simulink model "ES105A_StHlthSigNormn"  (R2013b)
settings: Solver=FixedStepDiscrete  SolverMode=SingleTasking  StartTime=0.0  StopTime=1  FixedStep=0.002  RelTol=1e-3
undefined symbols (not defined in the file): ARCHGLBPRM_FLOATZEROTHD_ULS_F32, CurrMeasCorrlnMaxErrCurr, CURRMOTSUMDIVBYZEROPROTNVAL_AMPR_F32, DIGTQDIVBYZEROPROTNVAL_HWNWTMTR_F32, DutyCycThermProtnDutyCycFildThd, EcuTMeasRngDiagcMax, EcuTMeasRngDiagcMin, EotLrngAuthyStrtLrn, FRICESTIMNDIVBYZEROPROTNVAL_HWNWTMTR_F32, HLTH0PERC_CNT_U08, HLTH100PERC_CNT_F32, HLTH100PERC_CNT_U08, HLTH50PERC_CNT_U08, HwTqCorrlnChATraSumSetFltThd, HwTqCorrlnChBTraSumSetFltThd, HWTQIDPTSIG_CNT_U08, MOTAG2MEAS_VALMAXERR_VOLTSQD_F32, MOTAG2MEAS_VALMINERR_VOLTSQD_F32, MOTAGCORRLN_MOTAGCORRLNERRTHD_MOTREVELEC_U0P16, MotDrvDiagcErrThd, MOTPOS2DIVBYZEROPROTNVAL2_VOLTSQD_F32, MOTPOS2DIVBYZEROPROTNVAL_VOLTSQD_F32, MOTPOSNERRDIVBYZEROPROTNVAL_MOTREV_U16, MOTPOSNERRZEROTHD_MOTREV_U0P16, NtcNr1, NtcSts1, PHAVLTGDIVBYZEROPROTNVAL_NANOSEC_F32, SigQlfr1, STHLTHSCAGFAC_CNT_F32, StHlthSigNormnAbsltMotPosDifStHlthDiagThd, StHlthSigNormnCurrMotSumStHlthDiagThd, StHlthSigNormnDigTqStHlthDiagThd, StHlthSigNormnDutyCycFltLimThd, StHlthSigNormnHiCtrlrT, StHlthSigNormnIdptSigStHlthSca, StHlthSigNormnLoCtrlrT, StHlthSigNormnMaxFricThd, StHlthSigNormnMinRackTrvlLim, StHlthSigNormnMotPosStHlthDiagThd, StHlthSigNormnMotVelCal, StHlthSigNormnPhaInfoStHlthDiagThd, StHlthSigNormnStHlthCorrlnErr, StHlthSigNormnStHlthCurrMotSum, StHlthSigNormnStHlthPhaInfo, StHlthSigNormnValMaxStHlthErr, StHlthSigNormnValMinStHlthErr, StHlthSigNormnWhlImbRejctnThd, SysGlbPrmMotPoleCnt, TSTHLTH0PERC_CNT_U08, u2, u3, u4, VLTGSTHLTH0PERC_CNT_U08
libraries: NxtrLim x39, simulink x33, NxtrAbslt x4
(part 8 of 10)

== system ES105A_StHlthSigNormn/StHlthSigNormn/UpdRawSig/Motor Position Error /AbsltMotPosABDifStHlth Calc/If Action Subsystem/If Action Subsystem1 ==
  MotAgABErrTerm : Inport
  Action Port : ActionPort  ActionType=else
  Constant3 : Constant  Value=STHLTHSCAGFAC_CNT_F32
  CopyRight2 : Subsystem  Description=|  mask(Copyright Information){none=on}
      | Copyright info block.                                               
      |                                                                     
      | Place copyright information at the top of every subsystem in design.
      mask prompts: none "No parameters"
      mask help: Place copyright information at the top of every subsystem in design.
      mask Display:
      | NxtrConf = 'Nexteer Confidential';
      | 
      | sys = bdroot; %handle for the current model ("system")
      | first = get_param(sys,'Created');
      | first = first(end-3:end);  %year is last four digits
      | 
      | last = get_param(sys,'LastModifiedDate');
      | if isempty(last)
      |     last = datestr(now,'yyyy');
      | else
      |     last = last(end-3:end);
      | end
      | 
      | if strcmp(first,last)
      |     fprintf('%s -- Copyright %s Nexteer',NxtrConf,first)
      | else
      |     fprintf('%s -- %s%s- %s Nexteer',NxtrConf,char(169),first,last)
      | end
  Data Store Read : DataStoreRead  DataStoreName=MotAgCorrlnErrThd
  Data Type Conversion : DataTypeConversion  OutDataTypeStr=uint8
  Divide : Product  Inputs=*/
  Divide by Zero Protection for Cal : Subsystem
  LimStat_f32 : NxtrLim/LimStat_f32  LoLim=STHLTHFLOATZEROVAL_ULS_F32  HiLim=STHLTHFLOATTWOFIFTYFIVEVAL_ULS_F32
      settings: AttributesFormatString=|
      | Low Limit: %<LoLim>
      | High Limit:%<HiLim>
  Product : Product
  Subtract : Sum  Inputs=+-
  AbsltMotPosABDiffStHlth : Outport
  wires:
  Data Store Read/1 -> Subtract/1
  Subtract/1 -> Divide/1
  Constant3/1 -> Product/2
  MotAgABErrTerm/1 -> Subtract/2
  Divide/1 -> Product/1
  Divide by Zero Protection for Cal/1(CorrlnDelta) -> Divide/2
  LimStat_f32/1 -> Data Type Conversion/1
  Data Type Conversion/1 -> AbsltMotPosABDiffStHlth/1
  Product/1 -> LimStat_f32/1

== system ES105A_StHlthSigNormn/StHlthSigNormn/UpdRawSig/Motor Position Error /AbsltMotPosABDifStHlth Calc/If Action Subsystem1/CopyRight2 ==

== system ES105A_StHlthSigNormn/StHlthSigNormn/UpdRawSig/Motor Position Error /AbsltMotPosACDifStHlth Calc/If Action Subsystem4/CopyRight2 ==

== system ES105A_StHlthSigNormn/StHlthSigNormn/UpdRawSig/Motor Position Error /AbsltMotPosACDifStHlth Calc/If Action Subsystem4/If Action Subsystem ==
  Action Port : ActionPort  ActionType=then
  Constant : Constant  Value=HLTH0PERC_CNT_U08  OutDataTypeStr=uint8
  CopyRight2 : Subsystem  Description=|  mask(Copyright Information){none=on}
      | Copyright info block.                                               
      |                                                                     
      | Place copyright information at the top of every subsystem in design.
      mask prompts: none "No parameters"
      mask help: Place copyright information at the top of every subsystem in design.
      mask Display:
      | NxtrConf = 'Nexteer Confidential';
      | 
      | sys = bdroot; %handle for the current model ("system")
      | first = get_param(sys,'Created');
      | first = first(end-3:end);  %year is last four digits
      | 
      | last = get_param(sys,'LastModifiedDate');
      | if isempty(last)
      |     last = datestr(now,'yyyy');
      | else
      |     last = last(end-3:end);
      | end
      | 
      | if strcmp(first,last)
      |     fprintf('%s -- Copyright %s Nexteer',NxtrConf,first)
      | else
      |     fprintf('%s -- %s%s- %s Nexteer',NxtrConf,char(169),first,last)
      | end
  AbsltMotPosACDiffStHlth : Outport
  wires:
  Constant/1 -> AbsltMotPosACDiffStHlth/1

== system ES105A_StHlthSigNormn/StHlthSigNormn/UpdRawSig/Motor Position Error /AbsltMotPosACDifStHlth Calc/If Action Subsystem4/If Action Subsystem1 ==
  MotAgACErrTerm : Inport
  Action Port : ActionPort  ActionType=else
  Constant3 : Constant  Value=STHLTHSCAGFAC_CNT_F32
  CopyRight2 : Subsystem  Description=|  mask(Copyright Information){none=on}
      | Copyright info block.                                               
      |                                                                     
      | Place copyright information at the top of every subsystem in design.
      mask prompts: none "No parameters"
      mask help: Place copyright information at the top of every subsystem in design.
      mask Display:
      | NxtrConf = 'Nexteer Confidential';
      | 
      | sys = bdroot; %handle for the current model ("system")
      | first = get_param(sys,'Created');
      | first = first(end-3:end);  %year is last four digits
      | 
      | last = get_param(sys,'LastModifiedDate');
      | if isempty(last)
      |     last = datestr(now,'yyyy');
      | else
      |     last = last(end-3:end);
      | end
      | 
      | if strcmp(first,last)
      |     fprintf('%s -- Copyright %s Nexteer',NxtrConf,first)
      | else
      |     fprintf('%s -- %s%s- %s Nexteer',NxtrConf,char(169),first,last)
      | end
  Data Store Read : DataStoreRead  DataStoreName=MotAgCorrlnErrThd
  Data Type Conversion : DataTypeConversion  OutDataTypeStr=uint8
  Divide : Product  Inputs=*/
  Divide by Zero Protection for Cal : Subsystem
  LimStat_f32 : NxtrLim/LimStat_f32  LoLim=STHLTHFLOATZEROVAL_ULS_F32  HiLim=STHLTHFLOATTWOFIFTYFIVEVAL_ULS_F32
      settings: AttributesFormatString=|
      | Low Limit: %<LoLim>
      | High Limit:%<HiLim>
  Product : Product
  Subtract : Sum  Inputs=+-
  AbsltMotPosACDiffStHlth : Outport
  wires:
  Data Store Read/1 -> Subtract/1
  Subtract/1 -> Divide/1
  Constant3/1 -> Product/2
  MotAgACErrTerm/1 -> Subtract/2
  Divide/1 -> Product/1
  Divide by Zero Protection for Cal/1(CorrlnDelta) -> Divide/2
  LimStat_f32/1 -> Data Type Conversion/1
  Product/1 -> LimStat_f32/1
  Data Type Conversion/1 -> AbsltMotPosACDiffStHlth/1

== system ES105A_StHlthSigNormn/StHlthSigNormn/UpdRawSig/Motor Position Error /AbsltMotPosACDifStHlth Calc/If Action Subsystem5/CopyRight2 ==

== system ES105A_StHlthSigNormn/StHlthSigNormn/UpdRawSig/Motor Position Error /AbsltMotPosBCDifStHlth Calc/If Action Subsystem8/CopyRight2 ==

== system ES105A_StHlthSigNormn/StHlthSigNormn/UpdRawSig/Motor Position Error /AbsltMotPosBCDifStHlth Calc/If Action Subsystem8/If Action Subsystem ==
  Action Port : ActionPort  ActionType=then
  Constant : Constant  Value=HLTH0PERC_CNT_U08  OutDataTypeStr=uint8
  CopyRight2 : Subsystem  Description=|  mask(Copyright Information){none=on}
      | Copyright info block.                                               
      |                                                                     
      | Place copyright information at the top of every subsystem in design.
      mask prompts: none "No parameters"
      mask help: Place copyright information at the top of every subsystem in design.
      mask Display:
      | NxtrConf = 'Nexteer Confidential';
      | 
      | sys = bdroot; %handle for the current model ("system")
      | first = get_param(sys,'Created');
      | first = first(end-3:end);  %year is last four digits
      | 
      | last = get_param(sys,'LastModifiedDate');
      | if isempty(last)
      |     last = datestr(now,'yyyy');
      | else
      |     last = last(end-3:end);
      | end
      | 
      | if strcmp(first,last)
      |     fprintf('%s -- Copyright %s Nexteer',NxtrConf,first)
      | else
      |     fprintf('%s -- %s%s- %s Nexteer',NxtrConf,char(169),first,last)
      | end
  AbsltMotPosBCDiffStHlth : Outport
  wires:
  Constant/1 -> AbsltMotPosBCDiffStHlth/1

== system ES105A_StHlthSigNormn/StHlthSigNormn/UpdRawSig/Motor Position Error /AbsltMotPosBCDifStHlth Calc/If Action Subsystem8/If Action Subsystem1 ==
  MotAgBCErrTerm : Inport
  Action Port : ActionPort  ActionType=else
  Constant3 : Constant  Value=STHLTHSCAGFAC_CNT_F32
  CopyRight2 : Subsystem  Description=|  mask(Copyright Information){none=on}
      | Copyright info block.                                               
      |                                                                     
      | Place copyright information at the top of every subsystem in design.
      mask prompts: none "No parameters"
      mask help: Place copyright information at the top of every subsystem in design.
      mask Display:
      | NxtrConf = 'Nexteer Confidential';
      | 
      | sys = bdroot; %handle for the current model ("system")
      | first = get_param(sys,'Created');
      | first = first(end-3:end);  %year is last four digits
      | 
      | last = get_param(sys,'LastModifiedDate');
      | if isempty(last)
      |     last = datestr(now,'yyyy');
      | else
      |     last = last(end-3:end);
      | end
      | 
      | if strcmp(first,last)
      |     fprintf('%s -- Copyright %s Nexteer',NxtrConf,first)
      | else
      |     fprintf('%s -- %s%s- %s Nexteer',NxtrConf,char(169),first,last)
      | end
  Data Store Read : DataStoreRead  DataStoreName=MotAgCorrlnErrThd
  Data Type Conversion : DataTypeConversion  OutDataTypeStr=uint8
  Divide : Product  Inputs=*/
  Divide by Zero Protection for Cal : Subsystem
  LimStat_f32 : NxtrLim/LimStat_f32  LoLim=STHLTHFLOATZEROVAL_ULS_F32  HiLim=STHLTHFLOATTWOFIFTYFIVEVAL_ULS_F32
      settings: AttributesFormatString=|
      | Low Limit: %<LoLim>
      | High Limit:%<HiLim>
  Product : Product
  Subtract : Sum  Inputs=+-
  AbsltMotPosBCDiffStHlth : Outport
  wires:
  Data Store Read/1 -> Subtract/1
  Subtract/1 -> Divide/1
  Constant3/1 -> Product/2
  MotAgBCErrTerm/1 -> Subtract/2
  Divide/1 -> Product/1
  Divide by Zero Protection for Cal/1(CorrlnDelta) -> Divide/2
  LimStat_f32/1 -> Data Type Conversion/1
  Data Type Conversion/1 -> AbsltMotPosBCDiffStHlth/1
  Product/1 -> LimStat_f32/1

== system ES105A_StHlthSigNormn/StHlthSigNormn/UpdRawSig/Motor Position Error /AbsltMotPosBCDifStHlth Calc/If Action Subsystem9/CopyRight2 ==

== system ES105A_StHlthSigNormn/StHlthSigNormn/UpdRawSig/Motor Position Error /AbsltMotPosPhaDifStHlth/SetNtcSts/CopyRight2 ==

== system ES105A_StHlthSigNormn/StHlthSigNormn/UpdRawSig/Motor Position Error /NTC Sts Calculation/NtcFaild/CopyRight2 ==

== system ES105A_StHlthSigNormn/StHlthSigNormn/UpdRawSig/Motor Position Error /NTC Sts Calculation/NtcPassd/CopyRight2 ==

== system ES105A_StHlthSigNormn/StHlthSigNormn/UpdRawSig/Phase Voltage Verification/NTC Sts Calculation/NtcFaild/CopyRight2 ==

== system ES105A_StHlthSigNormn/StHlthSigNormn/UpdRawSig/Phase Voltage Verification/NTC Sts Calculation/NtcPassd/CopyRight2 ==

== system ES105A_StHlthSigNormn/StHlthSigNormn/UpdRawSig/Phase Voltage Verification/PhaAStHlth Calc/If Action Subsystem/CopyRight2 ==

== system ES105A_StHlthSigNormn/StHlthSigNormn/UpdRawSig/Phase Voltage Verification/PhaAStHlth Calc/If Action Subsystem/If Action Subsystem ==
  Action Port : ActionPort  ActionType=then
  Constant : Constant  Value=HLTH0PERC_CNT_U08  OutDataTypeStr=uint8
  CopyRight2 : Subsystem  Description=|  mask(Copyright Information){none=on}
      | Copyright info block.                                               
      |                                                                     
      | Place copyright information at the top of every subsystem in design.
      mask prompts: none "No parameters"
      mask help: Place copyright information at the top of every subsystem in design.
      mask Display:
      | NxtrConf = 'Nexteer Confidential';
      | 
      | sys = bdroot; %handle for the current model ("system")
      | first = get_param(sys,'Created');
      | first = first(end-3:end);  %year is last four digits
      | 
      | last = get_param(sys,'LastModifiedDate');
      | if isempty(last)
      |     last = datestr(now,'yyyy');
      | else
      |     last = last(end-3:end);
      | end
      | 
      | if strcmp(first,last)
      |     fprintf('%s -- Copyright %s Nexteer',NxtrConf,first)
      | else
      |     fprintf('%s -- %s%s- %s Nexteer',NxtrConf,char(169),first,last)
      | end
  PhaseAStHlth : Outport
  wires:
  Constant/1 -> PhaseAStHlth/1

== system ES105A_StHlthSigNormn/StHlthSigNormn/UpdRawSig/Phase Voltage Verification/PhaAStHlth Calc/If Action Subsystem/If Action Subsystem1 ==
  MotDrvErrA : Inport
  Action Port : ActionPort  ActionType=else
  Constant : Constant  Value=MotDrvDiagcErrThd
  Constant3 : Constant  Value=STHLTHSCAGFAC_CNT_F32
  CopyRight2 : Subsystem  Description=|  mask(Copyright Information){none=on}
      | Copyright info block.                                               
      |                                                                     
      | Place copyright information at the top of every subsystem in design.
      mask prompts: none "No parameters"
      mask help: Place copyright information at the top of every subsystem in design.
      mask Display:
      | NxtrConf = 'Nexteer Confidential';
      | 
      | sys = bdroot; %handle for the current model ("system")
      | first = get_param(sys,'Created');
      | first = first(end-3:end);  %year is last four digits
      | 
      | last = get_param(sys,'LastModifiedDate');
      | if isempty(last)
      |     last = datestr(now,'yyyy');
      | else
      |     last = last(end-3:end);
      | end
      | 
      | if strcmp(first,last)
      |     fprintf('%s -- Copyright %s Nexteer',NxtrConf,first)
      | else
      |     fprintf('%s -- %s%s- %s Nexteer',NxtrConf,char(169),first,last)
      | end
  Data Type Conversion : DataTypeConversion  OutDataTypeStr=uint8
  Divide : Product  Inputs=*/
  Divide by Zero Protection for Cal : Subsystem
  LimStat_f32 : NxtrLim/LimStat_f32  LoLim=STHLTHFLOATZEROVAL_ULS_F32  HiLim=STHLTHFLOATTWOFIFTYFIVEVAL_ULS_F32
      settings: AttributesFormatString=|
      | Low Limit: %<LoLim>
      | High Limit:%<HiLim>
  Product : Product
  Subtract : Sum  Inputs=+-
  PhaseAStHlth : Outport
  wires:
  Constant/1 -> Subtract/1
  MotDrvErrA/1 -> Subtract/2
  Subtract/1 -> Divide/1
  Constant3/1 -> Product/2
  Divide/1 -> Product/1
  Divide by Zero Protection for Cal/1(MotDrvDiagDelta) -> Divide/2
  LimStat_f32/1 -> Data Type Conversion/1
  Product/1 -> LimStat_f32/1
  Data Type Conversion/1 -> PhaseAStHlth/1

== system ES105A_StHlthSigNormn/StHlthSigNormn/UpdRawSig/Phase Voltage Verification/PhaAStHlth Calc/If Action Subsystem1/CopyRight2 ==

== system ES105A_StHlthSigNormn/StHlthSigNormn/UpdRawSig/Phase Voltage Verification/PhaBStHlth Calc/If Action Subsystem4/CopyRight2 ==

== system ES105A_StHlthSigNormn/StHlthSigNormn/UpdRawSig/Phase Voltage Verification/PhaBStHlth Calc/If Action Subsystem4/If Action Subsystem ==
  Action Port : ActionPort  ActionType=then
  Constant : Constant  Value=HLTH0PERC_CNT_U08  OutDataTypeStr=uint8
  CopyRight2 : Subsystem  Description=|  mask(Copyright Information){none=on}
      | Copyright info block.                                               
      |                                                                     
      | Place copyright information at the top of every subsystem in design.
      mask prompts: none "No parameters"
      mask help: Place copyright information at the top of every subsystem in design.
      mask Display:
      | NxtrConf = 'Nexteer Confidential';
      | 
      | sys = bdroot; %handle for the current model ("system")
      | first = get_param(sys,'Created');
      | first = first(end-3:end);  %year is last four digits
      | 
      | last = get_param(sys,'LastModifiedDate');
      | if isempty(last)
      |     last = datestr(now,'yyyy');
      | else
      |     last = last(end-3:end);
      | end
      | 
      | if strcmp(first,last)
      |     fprintf('%s -- Copyright %s Nexteer',NxtrConf,first)
      | else
      |     fprintf('%s -- %s%s- %s Nexteer',NxtrConf,char(169),first,last)
      | end
  PhaseBStHlth : Outport
  wires:
  Constant/1 -> PhaseBStHlth/1

== system ES105A_StHlthSigNormn/StHlthSigNormn/UpdRawSig/Phase Voltage Verification/PhaBStHlth Calc/If Action Subsystem4/If Action Subsystem1 ==
  MotDrvErrB : Inport
  Action Port : ActionPort  ActionType=else
  Constant : Constant  Value=MotDrvDiagcErrThd
  Constant3 : Constant  Value=STHLTHSCAGFAC_CNT_F32
  CopyRight2 : Subsystem  Description=|  mask(Copyright Information){none=on}
      | Copyright info block.                                               
      |                                                                     
      | Place copyright information at the top of every subsystem in design.
      mask prompts: none "No parameters"
      mask help: Place copyright information at the top of every subsystem in design.
      mask Display:
      | NxtrConf = 'Nexteer Confidential';
      | 
      | sys = bdroot; %handle for the current model ("system")
      | first = get_param(sys,'Created');
      | first = first(end-3:end);  %year is last four digits
      | 
      | last = get_param(sys,'LastModifiedDate');
      | if isempty(last)
      |     last = datestr(now,'yyyy');
      | else
      |     last = last(end-3:end);
      | end
      | 
      | if strcmp(first,last)
      |     fprintf('%s -- Copyright %s Nexteer',NxtrConf,first)
      | else
      |     fprintf('%s -- %s%s- %s Nexteer',NxtrConf,char(169),first,last)
      | end
  Data Type Conversion : DataTypeConversion  OutDataTypeStr=uint8
  Divide : Product  Inputs=*/
  Divide by Zero Protection for Cal : Subsystem
  LimStat_f32 : NxtrLim/LimStat_f32  LoLim=STHLTHFLOATZEROVAL_ULS_F32  HiLim=STHLTHFLOATTWOFIFTYFIVEVAL_ULS_F32
      settings: AttributesFormatString=|
      | Low Limit: %<LoLim>
      | High Limit:%<HiLim>
  Product : Product
  Subtract : Sum  Inputs=+-
  PhaseBStHlth : Outport
  wires:
  Constant/1 -> Subtract/1
  MotDrvErrB/1 -> Subtract/2
  Subtract/1 -> Divide/1
  Constant3/1 -> Product/2
  Divide/1 -> Product/1
  Divide by Zero Protection for Cal/1(MotDrvDiagDelta) -> Divide/2
  LimStat_f32/1 -> Data Type Conversion/1
  Product/1 -> LimStat_f32/1
  Data Type Conversion/1 -> PhaseBStHlth/1

== system ES105A_StHlthSigNormn/StHlthSigNormn/UpdRawSig/Phase Voltage Verification/PhaBStHlth Calc/If Action Subsystem5/CopyRight2 ==

== system ES105A_StHlthSigNormn/StHlthSigNormn/UpdRawSig/Phase Voltage Verification/PhaCStHlth Calc/If Action Subsystem8/CopyRight2 ==

== system ES105A_StHlthSigNormn/StHlthSigNormn/UpdRawSig/Phase Voltage Verification/PhaCStHlth Calc/If Action Subsystem8/If Action Subsystem ==
  Action Port : ActionPort  ActionType=then
  Constant : Constant  Value=HLTH0PERC_CNT_U08  OutDataTypeStr=uint8
  CopyRight2 : Subsystem  Description=|  mask(Copyright Information){none=on}
      | Copyright info block.                                               
      |                                                                     
      | Place copyright information at the top of every subsystem in design.
      mask prompts: none "No parameters"
      mask help: Place copyright information at the top of every subsystem in design.
      mask Display:
      | NxtrConf = 'Nexteer Confidential';
      | 
      | sys = bdroot; %handle for the current model ("system")
      | first = get_param(sys,'Created');
      | first = first(end-3:end);  %year is last four digits
      | 
      | last = get_param(sys,'LastModifiedDate');
      | if isempty(last)
      |     last = datestr(now,'yyyy');
      | else
      |     last = last(end-3:end);
      | end
      | 
      | if strcmp(first,last)
      |     fprintf('%s -- Copyright %s Nexteer',NxtrConf,first)
      | else
      |     fprintf('%s -- %s%s- %s Nexteer',NxtrConf,char(169),first,last)
      | end
  PhaseCStHlth : Outport
  wires:
  Constant/1 -> PhaseCStHlth/1

== system ES105A_StHlthSigNormn/StHlthSigNormn/UpdRawSig/Phase Voltage Verification/PhaCStHlth Calc/If Action Subsystem8/If Action Subsystem1 ==
  MotDrvErrC : Inport
  Action Port : ActionPort  ActionType=else
  Constant : Constant  Value=MotDrvDiagcErrThd
  Constant3 : Constant  Value=STHLTHSCAGFAC_CNT_F32
  CopyRight2 : Subsystem  Description=|  mask(Copyright Information){none=on}
      | Copyright info block.                                               
      |                                                                     
      | Place copyright information at the top of every subsystem in design.
      mask prompts: none "No parameters"
      mask help: Place copyright information at the top of every subsystem in design.
      mask Display:
      | NxtrConf = 'Nexteer Confidential';
      | 
      | sys = bdroot; %handle for the current model ("system")
      | first = get_param(sys,'Created');
      | first = first(end-3:end);  %year is last four digits
      | 
      | last = get_param(sys,'LastModifiedDate');
      | if isempty(last)
      |     last = datestr(now,'yyyy');
      | else
      |     last = last(end-3:end);
      | end
      | 
      | if strcmp(first,last)
      |     fprintf('%s -- Copyright %s Nexteer',NxtrConf,first)
      | else
      |     fprintf('%s -- %s%s- %s Nexteer',NxtrConf,char(169),first,last)
      | end
  Data Type Conversion : DataTypeConversion  OutDataTypeStr=uint8
  Divide : Product  Inputs=*/
  Divide by Zero Protection for Cal : Subsystem
  LimStat_f32 : NxtrLim/LimStat_f32  LoLim=STHLTHFLOATZEROVAL_ULS_F32  HiLim=STHLTHFLOATTWOFIFTYFIVEVAL_ULS_F32
      settings: AttributesFormatString=|
      | Low Limit: %<LoLim>
      | High Limit:%<HiLim>
  Product : Product
  Subtract : Sum  Inputs=+-
  PhaseCStHlth : Outport
  wires:
  Constant/1 -> Subtract/1
  MotDrvErrC/1 -> Subtract/2
  Subtract/1 -> Divide/1
  Constant3/1 -> Product/2
  Divide/1 -> Product/1
  Divide by Zero Protection for Cal/1(MotDrvDiagDelta) -> Divide/2
  LimStat_f32/1 -> Data Type Conversion/1
  Product/1 -> LimStat_f32/1
  Data Type Conversion/1 -> PhaseCStHlth/1

== system ES105A_StHlthSigNormn/StHlthSigNormn/UpdRawSig/Phase Voltage Verification/PhaCStHlth Calc/If Action Subsystem9/CopyRight2 ==

== system ES105A_StHlthSigNormn/StHlthSigNormn/UpdRawSig/Phase Voltage Verification/PhaDStHlth Calc/If Action Subsystem12/CopyRight2 ==

== system ES105A_StHlthSigNormn/StHlthSigNormn/UpdRawSig/Phase Voltage Verification/PhaDStHlth Calc/If Action Subsystem12/If Action Subsystem ==
  Action Port : ActionPort  ActionType=then
  Constant : Constant  Value=HLTH0PERC_CNT_U08  OutDataTypeStr=uint8
  CopyRight2 : Subsystem  Description=|  mask(Copyright Information){none=on}
      | Copyright info block.                                               
      |                                                                     
      | Place copyright information at the top of every subsystem in design.
      mask prompts: none "No parameters"
      mask help: Place copyright information at the top of every subsystem in design.
      mask Display:
      | NxtrConf = 'Nexteer Confidential';
      | 
      | sys = bdroot; %handle for the current model ("system")
      | first = get_param(sys,'Created');
      | first = first(end-3:end);  %year is last four digits
      | 
      | last = get_param(sys,'LastModifiedDate');
      | if isempty(last)
      |     last = datestr(now,'yyyy');
      | else
      |     last = last(end-3:end);
      | end
      | 
      | if strcmp(first,last)
      |     fprintf('%s -- Copyright %s Nexteer',NxtrConf,first)
      | else
      |     fprintf('%s -- %s%s- %s Nexteer',NxtrConf,char(169),first,last)
      | end
  PhaseDStHlth : Outport
  wires:
  Constant/1 -> PhaseDStHlth/1

== system ES105A_StHlthSigNormn/StHlthSigNormn/UpdRawSig/Phase Voltage Verification/PhaDStHlth Calc/If Action Subsystem12/If Action Subsystem1 ==
  MotDrvErrD : Inport
  Action Port : ActionPort  ActionType=else
  Constant : Constant  Value=MotDrvDiagcErrThd
  Constant3 : Constant  Value=STHLTHSCAGFAC_CNT_F32
  CopyRight2 : Subsystem  Description=|  mask(Copyright Information){none=on}
      | Copyright info block.                                               
      |                                                                     
      | Place copyright information at the top of every subsystem in design.
      mask prompts: none "No parameters"
      mask help: Place copyright information at the top of every subsystem in design.
      mask Display:
      | NxtrConf = 'Nexteer Confidential';
      | 
      | sys = bdroot; %handle for the current model ("system")
      | first = get_param(sys,'Created');
      | first = first(end-3:end);  %year is last four digits
      | 
      | last = get_param(sys,'LastModifiedDate');
      | if isempty(last)
      |     last = datestr(now,'yyyy');
      | else
      |     last = last(end-3:end);
      | end
      | 
      | if strcmp(first,last)
      |     fprintf('%s -- Copyright %s Nexteer',NxtrConf,first)
      | else
      |     fprintf('%s -- %s%s- %s Nexteer',NxtrConf,char(169),first,last)
      | end
  Data Type Conversion : DataTypeConversion  OutDataTypeStr=uint8
  Divide : Product  Inputs=*/
  Divide by Zero Protection for Cal : Subsystem
  LimStat_f32 : NxtrLim/LimStat_f32  LoLim=STHLTHFLOATZEROVAL_ULS_F32  HiLim=STHLTHFLOATTWOFIFTYFIVEVAL_ULS_F32
      settings: AttributesFormatString=|
      | Low Limit: %<LoLim>
      | High Limit:%<HiLim>
  Product : Product
  Subtract : Sum  Inputs=+-
  PhaseDStHlth : Outport
  wires:
  Constant/1 -> Subtract/1
  MotDrvErrD/1 -> Subtract/2
  Subtract/1 -> Divide/1
  Constant3/1 -> Product/2
  Divide/1 -> Product/1
  Divide by Zero Protection for Cal/1(MotDrvDiagDelta) -> Divide/2
  LimStat_f32/1 -> Data Type Conversion/1
  Product/1 -> LimStat_f32/1
  Data Type Conversion/1 -> PhaseDStHlth/1

== system ES105A_StHlthSigNormn/StHlthSigNormn/UpdRawSig/Phase Voltage Verification/PhaDStHlth Calc/If Action Subsystem13/CopyRight2 ==

== system ES105A_StHlthSigNormn/StHlthSigNormn/UpdRawSig/Phase Voltage Verification/PhaEStHlth Calc/If Action Subsystem16/CopyRight2 ==

== system ES105A_StHlthSigNormn/StHlthSigNormn/UpdRawSig/Phase Voltage Verification/PhaEStHlth Calc/If Action Subsystem16/If Action Subsystem ==
  Action Port : ActionPort  ActionType=then
  Constant : Constant  Value=HLTH0PERC_CNT_U08  OutDataTypeStr=uint8
  CopyRight2 : Subsystem  Description=|  mask(Copyright Information){none=on}
      | Copyright info block.                                               
      |                                                                     
      | Place copyright information at the top of every subsystem in design.
      mask prompts: none "No parameters"
      mask help: Place copyright information at the top of every subsystem in design.
      mask Display:
      | NxtrConf = 'Nexteer Confidential';
      | 
      | sys = bdroot; %handle for the current model ("system")
      | first = get_param(sys,'Created');
      | first = first(end-3:end);  %year is last four digits
      | 
      | last = get_param(sys,'LastModifiedDate');
      | if isempty(last)
      |     last = datestr(now,'yyyy');
      | else
      |     last = last(end-3:end);
      | end
      | 
      | if strcmp(first,last)
      |     fprintf('%s -- Copyright %s Nexteer',NxtrConf,first)
      | else
      |     fprintf('%s -- %s%s- %s Nexteer',NxtrConf,char(169),first,last)
      | end
  PhaseEStHlth : Outport
  wires:
  Constant/1 -> PhaseEStHlth/1

== system ES105A_StHlthSigNormn/StHlthSigNormn/UpdRawSig/Phase Voltage Verification/PhaEStHlth Calc/If Action Subsystem16/If Action Subsystem1 ==
  MotDrvErrE : Inport
  Action Port : ActionPort  ActionType=else
  Constant : Constant  Value=MotDrvDiagcErrThd
  Constant3 : Constant  Value=STHLTHSCAGFAC_CNT_F32
  CopyRight2 : Subsystem  Description=|  mask(Copyright Information){none=on}
      | Copyright info block.                                               
      |                                                                     
      | Place copyright information at the top of every subsystem in design.
      mask prompts: none "No parameters"
      mask help: Place copyright information at the top of every subsystem in design.
      mask Display:
      | NxtrConf = 'Nexteer Confidential';
      | 
      | sys = bdroot; %handle for the current model ("system")
      | first = get_param(sys,'Created');
      | first = first(end-3:end);  %year is last four digits
      | 
      | last = get_param(sys,'LastModifiedDate');
      | if isempty(last)
      |     last = datestr(now,'yyyy');
      | else
      |     last = last(end-3:end);
      | end
      | 
      | if strcmp(first,last)
      |     fprintf('%s -- Copyright %s Nexteer',NxtrConf,first)
      | else
      |     fprintf('%s -- %s%s- %s Nexteer',NxtrConf,char(169),first,last)
      | end
  Data Type Conversion : DataTypeConversion  OutDataTypeStr=uint8
  Divide : Product  Inputs=*/
  Divide by Zero Protection for Cal : Subsystem
  LimStat_f32 : NxtrLim/LimStat_f32  LoLim=STHLTHFLOATZEROVAL_ULS_F32  HiLim=STHLTHFLOATTWOFIFTYFIVEVAL_ULS_F32
      settings: AttributesFormatString=|
      | Low Limit: %<LoLim>
      | High Limit:%<HiLim>
  Product : Product
  Subtract : Sum  Inputs=+-
  PhaseEStHlth : Outport
  wires:
  Constant/1 -> Subtract/1
  MotDrvErrE/1 -> Subtract/2
  Subtract/1 -> Divide/1
  Constant3/1 -> Product/2
  Divide/1 -> Product/1
  Divide by Zero Protection for Cal/1(MotDrvDiagDelta) -> Divide/2
  LimStat_f32/1 -> Data Type Conversion/1
  Product/1 -> LimStat_f32/1
  Data Type Conversion/1 -> PhaseEStHlth/1

== system ES105A_StHlthSigNormn/StHlthSigNormn/UpdRawSig/Phase Voltage Verification/PhaEStHlth Calc/If Action Subsystem17/CopyRight2 ==

== system ES105A_StHlthSigNormn/StHlthSigNormn/UpdRawSig/Phase Voltage Verification/PhaFStHlth Calc/If Action Subsystem20/CopyRight2 ==

== system ES105A_StHlthSigNormn/StHlthSigNormn/UpdRawSig/Phase Voltage Verification/PhaFStHlth Calc/If Action Subsystem20/If Action Subsystem ==
  Action Port : ActionPort  ActionType=then
  Constant : Constant  Value=HLTH0PERC_CNT_U08  OutDataTypeStr=uint8
  CopyRight2 : Subsystem  Description=|  mask(Copyright Information){none=on}
      | Copyright info block.                                               
      |                                                                     
      | Place copyright information at the top of every subsystem in design.
      mask prompts: none "No parameters"
      mask help: Place copyright information at the top of every subsystem in design.
      mask Display:
      | NxtrConf = 'Nexteer Confidential';
      | 
      | sys = bdroot; %handle for the current model ("system")
      | first = get_param(sys,'Created');
      | first = first(end-3:end);  %year is last four digits
      | 
      | last = get_param(sys,'LastModifiedDate');
      | if isempty(last)
      |     last = datestr(now,'yyyy');
      | else
      |     last = last(end-3:end);
      | end
      | 
      | if strcmp(first,last)
      |     fprintf('%s -- Copyright %s Nexteer',NxtrConf,first)
      | else
      |     fprintf('%s -- %s%s- %s Nexteer',NxtrConf,char(169),first,last)
      | end
  PhaseFStHlth : Outport
  wires:
  Constant/1 -> PhaseFStHlth/1

== system ES105A_StHlthSigNormn/StHlthSigNormn/UpdRawSig/Phase Voltage Verification/PhaFStHlth Calc/If Action Subsystem20/If Action Subsystem1 ==
  MotDrvErrF : Inport
  Action Port : ActionPort  ActionType=else
  Constant : Constant  Value=MotDrvDiagcErrThd
  Constant3 : Constant  Value=STHLTHSCAGFAC_CNT_F32
  CopyRight2 : Subsystem  Description=|  mask(Copyright Information){none=on}
      | Copyright info block.                                               
      |                                                                     
      | Place copyright information at the top of every subsystem in design.
      mask prompts: none "No parameters"
      mask help: Place copyright information at the top of every subsystem in design.
      mask Display:
      | NxtrConf = 'Nexteer Confidential';
      | 
      | sys = bdroot; %handle for the current model ("system")
      | first = get_param(sys,'Created');
      | first = first(end-3:end);  %year is last four digits
      | 
      | last = get_param(sys,'LastModifiedDate');
      | if isempty(last)
      |     last = datestr(now,'yyyy');
      | else
      |     last = last(end-3:end);
      | end
      | 
      | if strcmp(first,last)
      |     fprintf('%s -- Copyright %s Nexteer',NxtrConf,first)
      | else
      |     fprintf('%s -- %s%s- %s Nexteer',NxtrConf,char(169),first,last)
      | end
  Data Type Conversion : DataTypeConversion  OutDataTypeStr=uint8
  Divide : Product  Inputs=*/
  Divide by Zero Protection for Cal : Subsystem
  LimStat_f32 : NxtrLim/LimStat_f32  LoLim=STHLTHFLOATZEROVAL_ULS_F32  HiLim=STHLTHFLOATTWOFIFTYFIVEVAL_ULS_F32
      settings: AttributesFormatString=|
      | Low Limit: %<LoLim>
      | High Limit:%<HiLim>
  Product : Product
  Subtract : Sum  Inputs=+-
  PhaseFStHlth : Outport
  wires:
  Constant/1 -> Subtract/1
  MotDrvErrF/1 -> Subtract/2
  Subtract/1 -> Divide/1
  Constant3/1 -> Product/2
  Divide/1 -> Product/1
  Divide by Zero Protection for Cal/1(MotDrvDiagDelta) -> Divide/2
  LimStat_f32/1 -> Data Type Conversion/1
  Product/1 -> LimStat_f32/1
  Data Type Conversion/1 -> PhaseFStHlth/1

== system ES105A_StHlthSigNormn/StHlthSigNormn/UpdRawSig/Phase Voltage Verification/PhaFStHlth Calc/If Action Subsystem21/CopyRight2 ==

== system ES105A_StHlthSigNormn/StHlthSigNormn/UpdRawSig/Phase Voltage Verification/PhaStHlth/SetNtcSts/CopyRight2 ==

== system ES105A_StHlthSigNormn/StHlthSigNormn/UpdRawSig/ EOT Impact Counter/If Action Subsystem/If Action Subsystem/If Action Subsystem/CopyRight2 ==

== system ES105A_StHlthSigNormn/StHlthSigNormn/UpdRawSig/ EOT Impact Counter/If Action Subsystem/If Action Subsystem/If Action Subsystem/Do nothing ==
  note: Do Nothing
  Action Port : ActionPort  ActionType=else
  CopyRight2 : Subsystem  Description=|  mask(Copyright Information){none=on}
      | Copyright info block.                                               
      |                                                                     
      | Place copyright information at the top of every subsystem in design.
      mask prompts: none "No parameters"
      mask help: Place copyright information at the top of every subsystem in design.
      mask Display:
      | NxtrConf = 'Nexteer Confidential';
      | 
      | sys = bdroot; %handle for the current model ("system")
      | first = get_param(sys,'Created');
      | first = first(end-3:end);  %year is last four digits
      | 
      | last = get_param(sys,'LastModifiedDate');
      | if isempty(last)
      |     last = datestr(now,'yyyy');
      | else
      |     last = last(end-3:end);
      | end
      | 
      | if strcmp(first,last)
      |     fprintf('%s -- Copyright %s Nexteer',NxtrConf,first)
      | else
      |     fprintf('%s -- %s%s- %s Nexteer',NxtrConf,char(169),first,last)
      | end

== system ES105A_StHlthSigNormn/StHlthSigNormn/UpdRawSig/ EOT Impact Counter/If Action Subsystem/If Action Subsystem/If Action Subsystem/If Action Subsystem ==
  Action Port : ActionPort  ActionType=then
  CopyRight2 : Subsystem  Description=|  mask(Copyright Information){none=on}
      | Copyright info block.                                               
      |                                                                     
      | Place copyright information at the top of every subsystem in design.
      mask prompts: none "No parameters"
      mask help: Place copyright information at the top of every subsystem in design.
      mask Display:
      | NxtrConf = 'Nexteer Confidential';
      | 
      | sys = bdroot; %handle for the current model ("system")
      | first = get_param(sys,'Created');
      | first = first(end-3:end);  %year is last four digits
      | 
      | last = get_param(sys,'LastModifiedDate');
      | if isempty(last)
      |     last = datestr(now,'yyyy');
      | else
      |     last = last(end-3:end);
      | end
      | 
      | if strcmp(first,last)
      |     fprintf('%s -- Copyright %s Nexteer',NxtrConf,first)
      | else
      |     fprintf('%s -- %s%s- %s Nexteer',NxtrConf,char(169),first,last)
      | end
  Data Store Read : DataStoreRead  DataStoreName=EntrEot
  Do Nothing : Subsystem  TreatAsAtomicUnit=on
  If : If  IfExpression=u1
  If Action Subsystem : Subsystem  TreatAsAtomicUnit=on
  Logical Operator : Logic  Operator=NOT  Inputs=1  AllPortsSameDT=off  OutDataTypeStr=boolean
  wires:
  Data Store Read/1 -> Logical Operator/1
  If/1 -> If Action Subsystem/Action
  If/2 -> Do Nothing/Action
  Logical Operator/1 -> If/1

== system ES105A_StHlthSigNormn/StHlthSigNormn/UpdRawSig/ EOT Impact Counter/If Action Subsystem/If Action Subsystem/If Action Subsystem1/CopyRight2 ==

== system ES105A_StHlthSigNormn/StHlthSigNormn/UpdRawSig/ EOT Impact Counter/If Action Subsystem/If Action Subsystem1/If Action Subsystem/CopyRight2 ==

== system ES105A_StHlthSigNormn/StHlthSigNormn/UpdRawSig/ EOT Impact Counter/If Action Subsystem/If Action Subsystem1/If Action Subsystem/Do nothing ==
  note: Do Nothing
  Action Port : ActionPort  ActionType=else
  CopyRight2 : Subsystem  Description=|  mask(Copyright Information){none=on}
      | Copyright info block.                                               
      |                                                                     
      | Place copyright information at the top of every subsystem in design.
      mask prompts: none "No parameters"
      mask help: Place copyright information at the top of every subsystem in design.
      mask Display:
      | NxtrConf = 'Nexteer Confidential';
      | 
      | sys = bdroot; %handle for the current model ("system")
      | first = get_param(sys,'Created');
      | first = first(end-3:end);  %year is last four digits
      | 
      | last = get_param(sys,'LastModifiedDate');
      | if isempty(last)
      |     last = datestr(now,'yyyy');
      | else
      |     last = last(end-3:end);
      | end
      | 
      | if strcmp(first,last)
      |     fprintf('%s -- Copyright %s Nexteer',NxtrConf,first)
      | else
      |     fprintf('%s -- %s%s- %s Nexteer',NxtrConf,char(169),first,last)
      | end

== system ES105A_StHlthSigNormn/StHlthSigNormn/UpdRawSig/ EOT Impact Counter/If Action Subsystem/If Action Subsystem1/If Action Subsystem/If Action Subsystem ==
  Action Port : ActionPort  ActionType=then
  CopyRight2 : Subsystem  Description=|  mask(Copyright Information){none=on}
      | Copyright info block.                                               
      |                                                                     
      | Place copyright information at the top of every subsystem in design.
      mask prompts: none "No parameters"
      mask help: Place copyright information at the top of every subsystem in design.
      mask Display:
      | NxtrConf = 'Nexteer Confidential';
      | 
      | sys = bdroot; %handle for the current model ("system")
      | first = get_param(sys,'Created');
      | first = first(end-3:end);  %year is last four digits
      | 
      | last = get_param(sys,'LastModifiedDate');
      | if isempty(last)
      |     last = datestr(now,'yyyy');
      | else
      |     last = last(end-3:end);
      | end
      | 
      | if strcmp(first,last)
      |     fprintf('%s -- Copyright %s Nexteer',NxtrConf,first)
      | else
      |     fprintf('%s -- %s%s- %s Nexteer',NxtrConf,char(169),first,last)
      | end
  Data Store Read : DataStoreRead  DataStoreName=EntrEot
  Do nothing : Subsystem  TreatAsAtomicUnit=on
  If : If  IfExpression=u1
  If Action Subsystem : Subsystem  TreatAsAtomicUnit=on
  Logical Operator : Logic  Operator=NOT  Inputs=1  AllPortsSameDT=off  OutDataTypeStr=boolean
  wires:
  Data Store Read/1 -> Logical Operator/1
  If/1 -> If Action Subsystem/Action
  If/2 -> Do nothing/Action
  Logical Operator/1 -> If/1

== system ES105A_StHlthSigNormn/StHlthSigNormn/UpdRawSig/ EOT Impact Counter/If Action Subsystem/If Action Subsystem1/If Action Subsystem1/CopyRight2 ==

== system ES105A_StHlthSigNormn/StHlthSigNormn/UpdRawSig/Current Error/CurrMotSumABCStHlth Calc/If Action Subsystem/If Action Subsystem/CopyRight2 ==

== system ES105A_StHlthSigNormn/StHlthSigNormn/UpdRawSig/Current Error/CurrMotSumABCStHlth Calc/If Action Subsystem/If Action Subsystem1/CopyRight2 ==

== system ES105A_StHlthSigNormn/StHlthSigNormn/UpdRawSig/Current Error/CurrMotSumABCStHlth Calc/If Action Subsystem/If Action Subsystem1/Divide by Zero Protection for Cal ==
  Constant : Constant  Value=ARCHGLBPRM_FLOATZEROTHD_ULS_F32
  Constant1 : Constant  Value=StHlthSigNormnStHlthCurrMotSum
  Constant3 : Constant  Value=CurrMeasCorrlnMaxErrCurr
  CopyRight2 : Subsystem  Description=|  mask(Copyright Information){none=on}
      | Copyright info block.                                               
      |                                                                     
      | Place copyright information at the top of every subsystem in design.
      mask prompts: none "No parameters"
      mask help: Place copyright information at the top of every subsystem in design.
      mask Display:
      | NxtrConf = 'Nexteer Confidential';
      | 
      | sys = bdroot; %handle for the current model ("system")
      | first = get_param(sys,'Created');
      | first = first(end-3:end);  %year is last four digits
      | 
      | last = get_param(sys,'LastModifiedDate');
      | if isempty(last)
      |     last = datestr(now,'yyyy');
      | else
      |     last = last(end-3:end);
      | end
      | 
      | if strcmp(first,last)
      |     fprintf('%s -- Copyright %s Nexteer',NxtrConf,first)
      | else
      |     fprintf('%s -- %s%s- %s Nexteer',NxtrConf,char(169),first,last)
      | end
  If : If  IfExpression=u1
  If Zero : Subsystem  TreatAsAtomicUnit=on
  Merge : Merge
  Non Zero : Subsystem  TreatAsAtomicUnit=on
  Relational Operator : RelationalOperator  Operator=<=  OutDataTypeStr=boolean
  Subtract1 : Sum  Inputs=+-
  CurrMotSumDelta : Outport
  wires:
  If/1 -> If Zero/Action
  If/2 -> Non Zero/Action
  Subtract1/1 -> Non Zero/1(In1), Relational Operator/1
  If Zero/1(Out1) -> Merge/1
  Non Zero/1(Out1) -> Merge/2
  Merge/1 -> CurrMotSumDelta/1
  Relational Operator/1 -> If/1
  Constant/1 -> Relational Operator/2
  Constant3/1 -> Subtract1/1
  Constant1/1 -> Subtract1/2

== system ES105A_StHlthSigNormn/StHlthSigNormn/UpdRawSig/Current Error/CurrMotSumDEFStHlth Calc/If Action Subsystem4/If Action Subsystem/CopyRight2 ==

== system ES105A_StHlthSigNormn/StHlthSigNormn/UpdRawSig/Current Error/CurrMotSumDEFStHlth Calc/If Action Subsystem4/If Action Subsystem1/CopyRight2 ==

== system ES105A_StHlthSigNormn/StHlthSigNormn/UpdRawSig/Current Error/CurrMotSumDEFStHlth Calc/If Action Subsystem4/If Action Subsystem1/Divide by Zero Protection for Cal ==
  Constant : Constant  Value=ARCHGLBPRM_FLOATZEROTHD_ULS_F32
  Constant1 : Constant  Value=StHlthSigNormnStHlthCurrMotSum
  Constant3 : Constant  Value=CurrMeasCorrlnMaxErrCurr
  CopyRight2 : Subsystem  Description=|  mask(Copyright Information){none=on}
      | Copyright info block.                                               
      |                                                                     
      | Place copyright information at the top of every subsystem in design.
      mask prompts: none "No parameters"
      mask help: Place copyright information at the top of every subsystem in design.
      mask Display:
      | NxtrConf = 'Nexteer Confidential';
      | 
      | sys = bdroot; %handle for the current model ("system")
      | first = get_param(sys,'Created');
      | first = first(end-3:end);  %year is last four digits
      | 
      | last = get_param(sys,'LastModifiedDate');
      | if isempty(last)
      |     last = datestr(now,'yyyy');
      | else
      |     last = last(end-3:end);
      | end
      | 
      | if strcmp(first,last)
      |     fprintf('%s -- Copyright %s Nexteer',NxtrConf,first)
      | else
      |     fprintf('%s -- %s%s- %s Nexteer',NxtrConf,char(169),first,last)
      | end
  If : If  IfExpression=u1
  If Zero : Subsystem  TreatAsAtomicUnit=on
  Merge : Merge
  Non Zero : Subsystem  TreatAsAtomicUnit=on
  Relational Operator : RelationalOperator  Operator=<=  OutDataTypeStr=boolean
  Subtract1 : Sum  Inputs=+-
  CurrMotSumDelta : Outport
  wires:
  If/1 -> If Zero/Action
  If/2 -> Non Zero/Action
  Subtract1/1 -> Non Zero/1(In1), Relational Operator/1
  If Zero/1(Out1) -> Merge/1
  Non Zero/1(Out1) -> Merge/2
  Merge/1 -> CurrMotSumDelta/1
  Relational Operator/1 -> If/1
  Constant/1 -> Relational Operator/2
  Constant3/1 -> Subtract1/1
  Constant1/1 -> Subtract1/2

== system ES105A_StHlthSigNormn/StHlthSigNormn/UpdRawSig/Digital Torque Sensor /DigTqSnsrAStHlth Calc/If Action Subsystem1/Devide by Zero Protection for Cal/CopyRight2 ==

== system ES105A_StHlthSigNormn/StHlthSigNormn/UpdRawSig/Digital Torque Sensor /DigTqSnsrAStHlth Calc/If Action Subsystem1/Devide by Zero Protection for Cal/If Zero ==
  Action Port : ActionPort  ActionType=then
  Constant : Constant  Value=DIGTQDIVBYZEROPROTNVAL_HWNWTMTR_F32
  CopyRight2 : Subsystem  Description=|  mask(Copyright Information){none=on}
      | Copyright info block.                                               
      |                                                                     
      | Place copyright information at the top of every subsystem in design.
      mask prompts: none "No parameters"
      mask help: Place copyright information at the top of every subsystem in design.
      mask Display:
      | NxtrConf = 'Nexteer Confidential';
      | 
      | sys = bdroot; %handle for the current model ("system")
      | first = get_param(sys,'Created');
      | first = first(end-3:end);  %year is last four digits
      | 
      | last = get_param(sys,'LastModifiedDate');
      | if isempty(last)
      |     last = datestr(now,'yyyy');
      | else
      |     last = last(end-3:end);
      | end
      | 
      | if strcmp(first,last)
      |     fprintf('%s -- Copyright %s Nexteer',NxtrConf,first)
      | else
      |     fprintf('%s -- %s%s- %s Nexteer',NxtrConf,char(169),first,last)
      | end
  Out1 : Outport
  wires:
  Constant/1 -> Out1/1

== system ES105A_StHlthSigNormn/StHlthSigNormn/UpdRawSig/Digital Torque Sensor /DigTqSnsrAStHlth Calc/If Action Subsystem1/Devide by Zero Protection for Cal/Non Zero ==
  In1 : Inport
  Action Port : ActionPort  ActionType=else
  CopyRight2 : Subsystem  Description=|  mask(Copyright Information){none=on}
      | Copyright info block.                                               
      |                                                                     
      | Place copyright information at the top of every subsystem in design.
      mask prompts: none "No parameters"
      mask help: Place copyright information at the top of every subsystem in design.
      mask Display:
      | NxtrConf = 'Nexteer Confidential';
      | 
      | sys = bdroot; %handle for the current model ("system")
      | first = get_param(sys,'Created');
      | first = first(end-3:end);  %year is last four digits
      | 
      | last = get_param(sys,'LastModifiedDate');
      | if isempty(last)
      |     last = datestr(now,'yyyy');
      | else
      |     last = last(end-3:end);
      | end
      | 
      | if strcmp(first,last)
      |     fprintf('%s -- Copyright %s Nexteer',NxtrConf,first)
      | else
      |     fprintf('%s -- %s%s- %s Nexteer',NxtrConf,char(169),first,last)
      | end
  Out1 : Outport
  wires:
  In1/1 -> Out1/1

== system ES105A_StHlthSigNormn/StHlthSigNormn/UpdRawSig/Digital Torque Sensor /DigTqSnsrBStHlth Calc/If Action Subsystem3/Devide by Zero Protection for Cal/CopyRight2 ==
